simulink model "SG_GFOL_2020a"  (R2024a)
settings: Solver=ode1  StartTime=0.0  StopTime=Tsim  FixedStep=Ts  MaxStep=1e-4  RelTol=1e-4  EnableMultiTasking=on
values from neighbouring files (symbols this model uses):
  f1 = 50    [VSC_GF_SG_params.m]
  H = 5    [VSC_GF_SG_params.m]
  Inom_n2 = Sn_n2/Un_n2/sqrt(3)    [VSC_GF_SG_params.m]
  k_droop_f_n2 = 1/0.05    (= 20)    [VSC_GF_SG_params.m]
  ki_p_n2 = 1/tau_p    (= 5)    [VSC_GF_SG_params.m]
  ki_pll1 = kp_pll1/tau_pll_n1    [VSC_GF_SG_params.m]
  ki_pll_n2 = kp_pll_n2/tau_pll_n2    [VSC_GF_SG_params.m]
  ki_q_n2 = 1/tau_q    (= 5)    [VSC_GF_SG_params.m]
  ki_s_n2 = Rc_n2/taus_n2    (= 2048)    [VSC_GF_SG_params.m]
  kp_p_n2 = taus_n2/tau_p    (= 0.005)    [VSC_GF_SG_params.m]
  kp_pll1 = xi_pll_n1*2*omega_pll_n1/Vpeak    [VSC_GF_SG_params.m]
  kp_pll_n2 = xi_pll_n2*2*omega_pll_n2/Vpeak_n2    [VSC_GF_SG_params.m]
  kp_q_n2 = taus_n2/tau_q    (= 0.005)    [VSC_GF_SG_params.m]
  kp_s_n2 = Lc_n2/taus_n2    (= 130.379729381)    [VSC_GF_SG_params.m]
  Lac = Lpu*l*(Un1/Vl)^2    (= 0.105785123967)    [VSC_GF_SG_params.m]
  Lc_n2 = 0.2*Ln_n2    (= 0.130379729381)    [VSC_GF_SG_params.m]
  magnitud_delay = Ts    (= 5e-05)    [VSC_GF_SG_params.m]
  Pload_fnl = 400e6    (= 400000000)    [VSC_GF_SG_params.m]
  plots_step = Ts    (= 5e-05)    [VSC_GF_SG_params.m]
  Psg0_pu = Psg0/Pn    (= 0.4)    [VSC_GF_SG_params.m]
  Pvsc0 = Pload0 -Psg0    (= 200000000)    [VSC_GF_SG_params.m]
  Q_ref_n2 = 0e6    (= 0)    [VSC_GF_SG_params.m]
  Rac = Rpu*l*(Un1/Vl)^2    (= 3.17355371901)    [VSC_GF_SG_params.m]
  Rc_n2 = 0.01*Xn_n2    (= 2.048)    [VSC_GF_SG_params.m]
  Sn_n2 = Sn1    (= 500000000)    [VSC_GF_SG_params.m]
  Ssg = 500e6    (= 500000000)    [VSC_GF_SG_params.m]
  T_stp = 20    [VSC_GF_SG_params.m]
  tau_droop_fpll = 0.1    [VSC_GF_SG_params.m]
  tau_u = 40e-3    (= 0.04)    [VSC_GF_SG_params.m]
  Ts = 5e-5    (= 5e-05)    [VSC_GF_SG_params.m]
  Tsim = 40    [VSC_GF_SG_params.m]
  Un1 = 320e3    (= 320000)    [VSC_GF_SG_params.m]
  Vdcref_n1 = 640e3    (= 640000)    [VSC_GF_SG_params.m]
  Vpeak = Un1*sqrt(2/3)    [VSC_GF_SG_params.m]
  Vpeak_n1 = Un_n1/sqrt(3)*sqrt(2)    [VSC_GF_SG_params.m]
  Vpeak_n2 = Un_n2/sqrt(3)*sqrt(2)    [VSC_GF_SG_params.m]
  w_g1 = 2*pi*f1    (= 314.159265359)    [VSC_GF_SG_params.m]
  w_n2 = 2*pi*f_n2    (= 314.159265359)    [VSC_GF_SG_params.m]
undefined symbols (not defined in the file or in its folder): D11, Delta, k, magnitude, P_set, P_step, Pload_init, Q_set, Q_step, t_ramp, t_step_P, t_step_Q, tau_ramp, tau_wf
libraries: simulink x6, simulink_extras x6, spsSeriesRLCBranchLib x6, spsThreePhaseParallelRLCLoadLib x4, spsControlledVoltageSourceLib x4, spsCurrentMeasurementLib x4, spsControlledCurrentSourceLib x3, spsVoltageMeasurementLib x3, spsLoadFlowBusLib x2, slpidlib x2, spsGroundLib x2, spsSampleandHoldLib x1
(part 2 of 2)

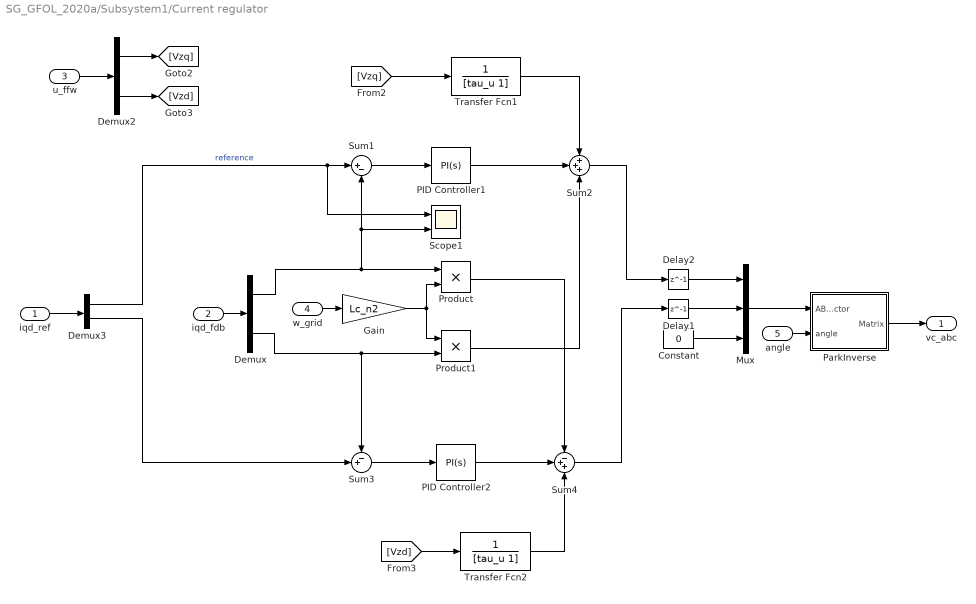
== system SG_GFOL_2020a/Subsystem1/Current regulator ==
  iqd_ref : Inport
  iqd_fdb : Inport  Port=2
  u_ffw : Inport  Port=3
  w_grid : Inport  Port=4
  angle : Inport  Port=5
  Constant : Constant  Value=0
  Delay1 : Delay  DelayLength=1  InitialCondition=0  SampleTime=magnitud_delay
  Delay2 : Delay  DelayLength=1  InitialCondition=Vpeak  SampleTime=magnitud_delay
  Demux : Demux  Outputs=2
  Demux2 : Demux  Outputs=2
  Demux3 : Demux  Outputs=2
  Gain : Gain  Gain=Lc_n2
  Mux : Mux  Inputs=3
  PID Controller1 : slpidlib/PID Controller  Controller=PI  Form=Parallel  TimeDomain=Continuous-time  UseExternalTs=off  SampleTime=-1  IntegratorMethod=Forward Euler  FilterMethod=Forward Euler  ControllerParametersSource=internal  P=kp_s_n2  I=ki_s_n2  UseKiTs=off  D=0  UseExternalDerivativeSource=off  N=100  UseFilter=on  TunerSelectOption=Transfer Function Based (PID Tuner App)  InitialConditionSource=internal  InitialConditionForIntegrator=0  InitialConditionForFilter=0  DifferentiatorICPrevScaledInput=0  ExternalReset=none  TrackingMode=off  Kt=1  LimitOutput=off  SatLimitsSource=internal  UpperSaturationLimit=inf  LowerSaturationLimit=-inf  LinearizeAsGain=on  AntiWindupMode=none  Kb=1  LimitIntegrator=off  UpperIntegratorSaturationLimit=inf  LowerIntegratorSaturationLimit=-inf  POutMin=[]  POutMax=[]  IOutMin=[]  IOutMax=[]  DOutMin=[]  DOutMax=[]  NOutMin=[]  NOutMax=[]  SumOutMin=[]  SumOutMax=[]  SaturationOutMin=[]  SaturationOutMax=[]  PParamMin=[]  PParamMax=[]  IParamMin=[]  IParamMax=[]  DParamMin=[]  DParamMax=[]  NParamMin=[]  NParamMax=[]  KbParamMin=[]  KbParamMax=[]  KtParamMin=[]  KtParamMax=[]  KbOutMin=[]  KbOutMax=[]  KtOutMin=[]  KtOutMax=[]  IntegratorOutMin=[]  IntegratorOutMax=[]  FilterOutMin=[]  FilterOutMax=[]  SumI1OutMin=[]  SumI1OutMax=[]  SumI2OutMin=[]  SumI2OutMax=[]  SumI3OutMin=[]  SumI3OutMax=[]  SumI4OutMin=[]  SumI4OutMax=[]  SumDOutMin=[]  SumDOutMax=[]  DifferentiatorOutMin=[]  DifferentiatorOutMax=[]  FilterDiffOutCoefMin=[]  FilterDiffOutCoefMax=[]  ReciprocalOutMin=[]  ReciprocalOutMax=[]  SumDenOutMin=[]  SumDenOutMax=[]  SumNumOutMin=[]  SumNumOutMax=[]  DivideOutMin=[]  DivideOutMax=[]  UdiffTsProdOutMin=[]  UdiffTsProdOutMax=[]  NTsProdOutMin=[]  NTsProdOutMax=[]  UintegralTsProdOutMin=[]  UintegralTsProdOutMax=[]  UngainTsProdOutMin=[]  UngainTsProdOutMax=[]  ClampingZeroOutDataTypeStr=Inherit: Inherit via back propagation  ClampingZeroOutMin=[]  ClampingZeroOutMax=[]  FilterDenConstantOutDataTypeStr=Inherit: Inherit via back propagation  FilterDenConstantOutMin=[]  FilterDenConstantOutMax=[]  PCopyOutDataTypeStr=Inherit: Inherit via back propagation  PCopyOutMin=[]  PCopyOutMax=[]  NCopyOutDataTypeStr=Inherit: Inherit via back propagation  NCopyOutMin=[]  NCopyOutMax=[]  IntegratorContinuousStateAttributes=''  IntegratorStateMustResolveToSignalObject=off  IntegratorRTWStateStorageClass=Auto  FilterContinuousStateAttributes=''  FilterStateMustResolveToSignalObject=off  FilterRTWStateStorageClass=Auto  ParallelPVariant=InternalParameters  IdealPVariant=Disabled  IVariant=InternalParameters  DVariant=Disabled  IntegratorVariant=Continuous  SatVariant=Disabled  AWVariant=Passthrough  PCopyVariant=Disabled  TRVariant=Disabled  FdbkBlocksVariant=Forward  IdealPFdbkVariant=Disabled  SatFdbkVariant=Disabled  DerivativeFilterVariant=Disabled  NVariant=Disabled  NCopyVariant=Disabled_SignalSpec  FilterICVariant=Disabled  IntegratorICVariant=InternalICs  ExternalResetVariant=Disabled  TRSumVariant=Passthrough  SumFdbkVariant=Disabled  SumVariant=Sum_PI  TsampFilterVariant=InternalTs  TsampNgainVariant=Passthrough  TsampIntegralVariant=Disabled_SignalSpec  ExternalSaturationOutDataTypeStr=Inherit: Same as second input  DerivativeSourceVariant=Disabled
  PID Controller2 : slpidlib/PID Controller  Controller=PI  Form=Parallel  TimeDomain=Continuous-time  UseExternalTs=off  SampleTime=-1  IntegratorMethod=Forward Euler  FilterMethod=Forward Euler  ControllerParametersSource=internal  P=kp_s_n2  I=ki_s_n2  UseKiTs=off  D=0  UseExternalDerivativeSource=off  N=100  UseFilter=on  TunerSelectOption=Transfer Function Based (PID Tuner App)  InitialConditionSource=internal  InitialConditionForIntegrator=0  InitialConditionForFilter=0  DifferentiatorICPrevScaledInput=0  ExternalReset=none  TrackingMode=off  Kt=1  LimitOutput=off  SatLimitsSource=internal  UpperSaturationLimit=inf  LowerSaturationLimit=-inf  LinearizeAsGain=on  AntiWindupMode=none  Kb=1  LimitIntegrator=off  UpperIntegratorSaturationLimit=inf  LowerIntegratorSaturationLimit=-inf  POutMin=[]  POutMax=[]  IOutMin=[]  IOutMax=[]  DOutMin=[]  DOutMax=[]  NOutMin=[]  NOutMax=[]  SumOutMin=[]  SumOutMax=[]  SaturationOutMin=[]  SaturationOutMax=[]  PParamMin=[]  PParamMax=[]  IParamMin=[]  IParamMax=[]  DParamMin=[]  DParamMax=[]  NParamMin=[]  NParamMax=[]  KbParamMin=[]  KbParamMax=[]  KtParamMin=[]  KtParamMax=[]  KbOutMin=[]  KbOutMax=[]  KtOutMin=[]  KtOutMax=[]  IntegratorOutMin=[]  IntegratorOutMax=[]  FilterOutMin=[]  FilterOutMax=[]  SumI1OutMin=[]  SumI1OutMax=[]  SumI2OutMin=[]  SumI2OutMax=[]  SumI3OutMin=[]  SumI3OutMax=[]  SumI4OutMin=[]  SumI4OutMax=[]  SumDOutMin=[]  SumDOutMax=[]  DifferentiatorOutMin=[]  DifferentiatorOutMax=[]  FilterDiffOutCoefMin=[]  FilterDiffOutCoefMax=[]  ReciprocalOutMin=[]  ReciprocalOutMax=[]  SumDenOutMin=[]  SumDenOutMax=[]  SumNumOutMin=[]  SumNumOutMax=[]  DivideOutMin=[]  DivideOutMax=[]  UdiffTsProdOutMin=[]  UdiffTsProdOutMax=[]  NTsProdOutMin=[]  NTsProdOutMax=[]  UintegralTsProdOutMin=[]  UintegralTsProdOutMax=[]  UngainTsProdOutMin=[]  UngainTsProdOutMax=[]  ClampingZeroOutDataTypeStr=Inherit: Inherit via back propagation  ClampingZeroOutMin=[]  ClampingZeroOutMax=[]  FilterDenConstantOutDataTypeStr=Inherit: Inherit via back propagation  FilterDenConstantOutMin=[]  FilterDenConstantOutMax=[]  PCopyOutDataTypeStr=Inherit: Inherit via back propagation  PCopyOutMin=[]  PCopyOutMax=[]  NCopyOutDataTypeStr=Inherit: Inherit via back propagation  NCopyOutMin=[]  NCopyOutMax=[]  IntegratorContinuousStateAttributes=''  IntegratorStateMustResolveToSignalObject=off  IntegratorRTWStateStorageClass=Auto  FilterContinuousStateAttributes=''  FilterStateMustResolveToSignalObject=off  FilterRTWStateStorageClass=Auto  ParallelPVariant=InternalParameters  IdealPVariant=Disabled  IVariant=InternalParameters  DVariant=Disabled  IntegratorVariant=Continuous  SatVariant=Disabled  AWVariant=Passthrough  PCopyVariant=Disabled  TRVariant=Disabled  FdbkBlocksVariant=Forward  IdealPFdbkVariant=Disabled  SatFdbkVariant=Disabled  DerivativeFilterVariant=Disabled  NVariant=Disabled  NCopyVariant=Disabled_SignalSpec  FilterICVariant=Disabled  IntegratorICVariant=InternalICs  ExternalResetVariant=Disabled  TRSumVariant=Passthrough  SumFdbkVariant=Disabled  SumVariant=Sum_PI  TsampFilterVariant=InternalTs  TsampNgainVariant=Passthrough  TsampIntegralVariant=Disabled_SignalSpec  ExternalSaturationOutDataTypeStr=Inherit: Same as second input  DerivativeSourceVariant=Disabled
  ParkInverse : Subsystem  mask(Gerard){}
      mask help:
      | This block applies the park inverse transfomation from a desired vector.
      | The input Xqd0 refers to the vector in the qd0 frame, and the second input is the angle used in the inverse transformation.
      | The output is the vector in the ABC frame.
      mask Display:
      | port_label('output',1,'Xabc')
      | port_label('input',1,'Xqd0')
      | port_label('input',2,'angle')
  Product : Product  RndMeth=Zero
  Product1 : Product  RndMeth=Zero
  Scope1 : Scope  NumInputPorts=2
  Sum1 : Sum  Inputs=|+-
  Sum2 : Sum  Inputs=+++
  Sum3 : Sum  Inputs=-+|
  Sum4 : Sum  Inputs=-++
  Transfer Fcn1 : TransferFcn  Denominator=[tau_u 1]
  Transfer Fcn2 : TransferFcn  Denominator=[tau_u 1]
  vc_abc : Outport
  wires:
  Transfer Fcn2/1 -> Sum4/3
  [Vzq] -> Transfer Fcn1/1
  Demux3/2 -> Sum3/2
  iqd_ref/1 -> Demux3/1
  Demux3/1 -> Scope1/1, Sum1/1  "reference"
  PID Controller2/1 -> Sum4/2
  Sum3/1 -> PID Controller2/1
  Sum1/1 -> PID Controller1/1
  angle/1 -> ParkInverse/2(angle)
  [Vzd] -> Transfer Fcn2/1
  u_ffw/1 -> Demux2/1
  Demux2/2 -> [Vzd]
  Demux2/1 -> [Vzq]
  Mux/1 -> ParkInverse/1(ABC vector)
  Transfer Fcn1/1 -> Sum2/1
  ParkInverse/1(Matrix) -> vc_abc/1
  Constant/1 -> Mux/3
  Product/1 -> Sum4/1
  Product1/1 -> Sum2/3
  Demux/2 -> Sum3/1, Product1/2
  Gain/1 -> Product/2, Product1/1
  Demux/1 -> Product/1, Scope1/2, Sum1/2
  PID Controller1/1 -> Sum2/2
  w_grid/1 -> Gain/1
  iqd_fdb/1 -> Demux/1
  Sum4/1 -> Delay1/1
  Sum2/1 -> Delay2/1
  Delay1/1 -> Mux/2
  Delay2/1 -> Mux/1

== system SG_GFOL_2020a/Subsystem1/Frequency support ==
  wref : Inport
  wpll : Inport  Port=2
  Pref0 : Inport  Port=3
  Gain1 : Gain  Gain=Sn_n2
  Gain10 : Gain  Gain=1/w_n2
  Product : Product
  Sum2 : Sum  Inputs=|+-
  Sum3 : Sum  Inputs=|++
  Transfer Fcn2 : TransferFcn  Denominator=[tau_droop_fpll 1]
  kdroop : Step  After=k_droop_f_n2  SampleTime=0
  Pref : Outport
  wires:
  Gain1/1 -> Sum3/1
  Gain10/1 -> Product/1
  Transfer Fcn2/1 -> Sum2/2
  kdroop/1 -> Product/2
  Product/1 -> Gain1/1
  wpll/1 -> Transfer Fcn2/1
  Sum3/1 -> Pref/1
  Pref0/1 -> Sum3/2
  Sum2/1 -> Gain10/1
  wref/1 -> Sum2/1

== system SG_GFOL_2020a/Subsystem1/PLL ==
  Vabc : Inport
  Constant1 : Constant  Value=w_n2
  Demux3 : Demux  Outputs=3
  Integrator2 : Integrator
  Integrator3 : Integrator
  Mux : Mux  Inputs=2
  ParkTransform4 : Subsystem  mask(Gerard){}
      mask help:
      | This block applies the park transfomation from a desired vector.
      | The input Xabc refers to the vector in the ABC frame, and the second input is the angle used in the transformation.
      | The output is the vector in the qd0 frame.
      mask Display:
      | port_label('output',1,'Xqd0')
      | port_label('input',1,'Xabc')
      | port_label('input',2,'angle')
  Sum1 : Sum  Inputs=+++
  Terminator : Terminator
  ki1 : Gain  Gain=ki_pll_n2
  kp1 : Gain  Gain=-1
  kp2 : Gain  Gain=kp_pll_n2
  omega : Outport  VectorParamsAs1DForOutWhenUnconnected=off
  angle : Outport  Port=2  VectorParamsAs1DForOutWhenUnconnected=off
  vqd : Outport  Port=3  VectorParamsAs1DForOutWhenUnconnected=off
  wires:
  Sum1/1 -> omega/1, Integrator3/1
  Demux3/1 -> Mux/1
  Constant1/1 -> Sum1/1
  ki1/1 -> Integrator2/1
  kp1/1 -> kp2/1, ki1/1
  Integrator2/1 -> Sum1/3
  kp2/1 -> Sum1/2
  Integrator3/1 -> ParkTransform4/2(angle), angle/1
  Demux3/2 -> Mux/2, kp1/1  "Vd"
  Vabc/1 -> ParkTransform4/1(ABC vector)
  ParkTransform4/1(Matrix) -> Demux3/1
  Demux3/3 -> Terminator/1
  Mux/1 -> vqd/1

== system SG_GFOL_2020a/Subsystem1/PQ Calculation1 ==
  u_qd : Inport
  ig_qd : Inport  Port=2
  Add1 : Sum  Inputs=-+
  Add2 : Sum
  Demux4 : Demux  Outputs=2
  Demux7 : Demux  Outputs=2
  Gain1 : Gain  Gain=3/2
  Gain12 : Gain  Gain=3/2
  Product{,1..3} (4 alike) : Product
  P : Outport
  Q : Outport  Port=2
  wires:
  Gain12/1 -> P/1
  Gain1/1 -> Q/1
  u_qd/1 -> Demux7/1
  ig_qd/1 -> Demux4/1
  Product3/1 -> Add1/2
  Add1/1 -> Gain1/1
  Demux4/1 -> Product/2, Product2/2
  Product2/1 -> Add1/1
  Demux7/1 -> Product/1, Product3/1
  Add2/1 -> Gain12/1
  Product1/1 -> Add2/2
  Product/1 -> Add2/1
  Demux7/2 -> Product1/1, Product2/1
  Demux4/2 -> Product3/2, Product1/2

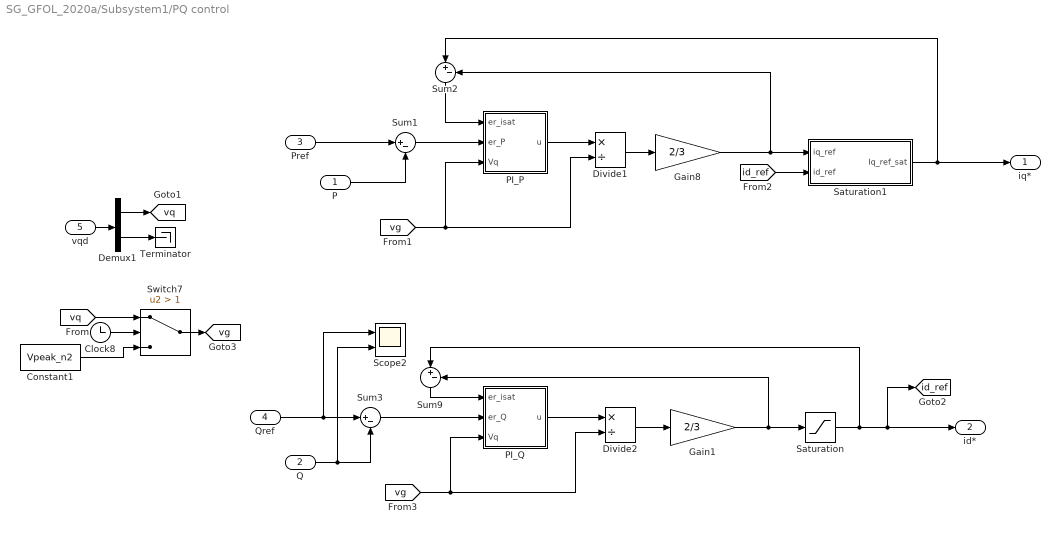
== system SG_GFOL_2020a/Subsystem1/PQ control ==
  P : Inport
  Q : Inport  Port=2
  Pref : Inport  Port=3
  Qref : Inport  Port=4
  vqd : Inport  Port=5
  Clock8 : Clock
  Constant1 : Constant  Value=Vpeak_n2
  Demux1 : Demux  Outputs=2
  Divide1 : Product  Inputs=*/
  Divide2 : Product  Inputs=*/
  Gain1 : Gain  Gain=2/3
  Gain8 : Gain  Gain=2/3
  PI_P : Subsystem
  PI_Q : Subsystem
  Saturation : Saturate  UpperLimit=Inom_n2  LowerLimit=-Inom_n2
  Saturation1 : Subsystem
  Scope2 : Scope  NumInputPorts=2
  Sum{1..3,9} (4 alike) : Sum  Inputs=|+-
  Switch7 : Switch  Criteria=u2 > Threshold  Threshold=1  SaturateOnIntegerOverflow=off  InputSameDT=off
  Terminator : Terminator
  iq* : Outport
  id* : Outport  Port=2
  tag scope: id_ref=global, vg=global, vq=global
  wires:
  Gain1/1 -> Sum9/2, Saturation/1
  Pref/1 -> Sum1/1
  Sum3/1 -> PI_Q/2(er_Q)
  Qref/1 -> Scope2/1, Sum3/1
  P/1 -> Sum1/2
  Q/1 -> Scope2/2, Sum3/2
  [vg] -> Divide1/2, PI_P/3(Vq)
  PI_P/1(u) -> Divide1/1
  Gain8/1 -> Sum2/2, Saturation1/1(iq_ref)
  Saturation1/1(Iq_ref_sat) -> Sum2/1, iq*/1
  Divide1/1 -> Gain8/1
  Sum1/1 -> PI_P/2(er_P)
  vqd/1 -> Demux1/1
  Demux1/2 -> Terminator/1
  PI_Q/1(u) -> Divide2/1
  Divide2/1 -> Gain1/1
  Demux1/1 -> [vq]
  [vg] -> PI_Q/3(Vq), Divide2/2
  Saturation/1 -> [id_ref], id*/1, Sum9/1
  Sum9/1 -> PI_Q/1(er_isat)
  Sum2/1 -> PI_P/1(er_isat)
  [id_ref] -> Saturation1/2(id_ref)
  [vq] -> Switch7/1
  Constant1/1 -> Switch7/3
  Clock8/1 -> Switch7/2
  Switch7/1 -> [vg]

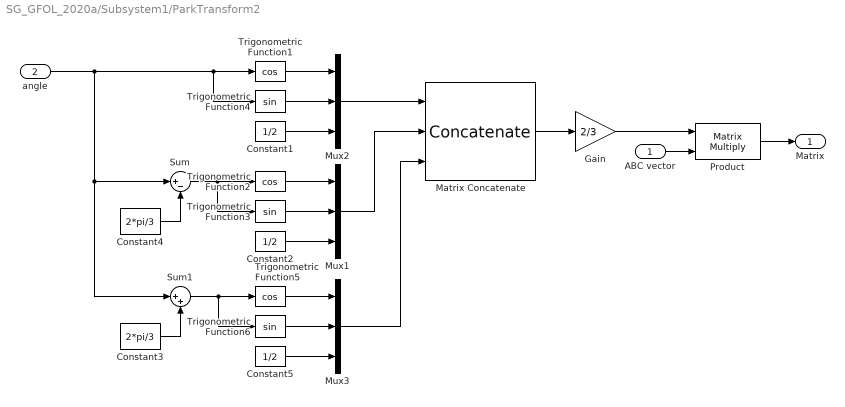
== system SG_GFOL_2020a/Subsystem1/ParkTransform2 ==
  ABC vector : Inport
  angle : Inport  Port=2
  Constant1 : Constant  Value=1/2
  Constant2 : Constant  Value=1/2
  Constant3 : Constant  Value=2*pi/3
  Constant4 : Constant  Value=2*pi/3
  Constant5 : Constant  Value=1/2
  Gain : Gain  Gain=2/3
  Matrix Concatenate : Concatenate  NumInputs=3  Mode=Multidimensional array  ConcatenateDimension=2
  Mux1 : Mux  Inputs=3
  Mux2 : Mux  Inputs=3
  Mux3 : Mux  Inputs=3
  Product : Product  Multiplication=Matrix(*)  RndMeth=Zero
  Sum : Sum  Inputs=|+-
  Sum1 : Sum  Inputs=|++
  Trigonometric Function1 : Trigonometry  Operator=cos
  Trigonometric Function2 : Trigonometry  Operator=cos
  Trigonometric Function3 : Trigonometry
  Trigonometric Function4 : Trigonometry
  Trigonometric Function5 : Trigonometry  Operator=cos
  Trigonometric Function6 : Trigonometry
  Matrix : Outport
  wires:
  Mux3/1 -> Matrix Concatenate/3
  Mux2/1 -> Matrix Concatenate/1
  Mux1/1 -> Matrix Concatenate/2
  Sum1/1 -> Trigonometric Function5/1, Trigonometric Function6/1
  Constant5/1 -> Mux3/3
  Trigonometric Function5/1 -> Mux3/1
  Trigonometric Function6/1 -> Mux3/2
  Constant1/1 -> Mux2/3
  Trigonometric Function1/1 -> Mux2/1
  Trigonometric Function4/1 -> Mux2/2
  Sum/1 -> Trigonometric Function2/1, Trigonometric Function3/1
  Constant2/1 -> Mux1/3
  Trigonometric Function2/1 -> Mux1/1
  Trigonometric Function3/1 -> Mux1/2
  angle/1 -> Sum/1, Sum1/1, Trigonometric Function1/1, Trigonometric Function4/1
  Constant3/1 -> Sum1/2
  Constant4/1 -> Sum/2
  Gain/1 -> Product/1
  Product/1 -> Matrix/1
  ABC vector/1 -> Product/2
  Matrix Concatenate/1 -> Gain/1

== system SG_GFOL_2020a/Subsystem1/VSC n1 ==
  vc_abc : Inport
  i_abc : Inport  Port=2
  Vbus : Inport  Port=3
  Controlled Current Source5 : spsControlledCurrentSourceLib/Controlled Current Source  Initialize=on  Source_Type=DC  Amplitude=0  Phase=0  Frequency=0  Measurements=None
  Controlled Voltage Source1 : spsControlledVoltageSourceLib/Controlled Voltage Source  Initialize=off  Source_Type=AC  Amplitude=0  Phase=0  Frequency=0  Measurements=None
  Controlled Voltage Source2 : spsControlledVoltageSourceLib/Controlled Voltage Source  Initialize=off  Source_Type=AC  Amplitude=0  Phase=0  Frequency=0  Measurements=None
  Controlled Voltage Source3 : spsControlledVoltageSourceLib/Controlled Voltage Source  Initialize=off  Source_Type=AC  Amplitude=0  Phase=0  Frequency=0  Measurements=None
  Current Measurement9 : spsCurrentMeasurementLib/Current Measurement  PhasorSimulation=off  OutputType=Complex  PSBequivalent=0
  Demux : Demux  Outputs=3
  Divide : Product  Inputs=*/
  Ground : spsGroundLib/Ground  LConnTagsString=a
  Product1 : Product  InputSameDT=on  SaturateOnIntegerOverflow=on  OutDataTypeStr=Inherit: Same as first input
  Sum4 : Sum  Inputs=1  InputSameDT=on  SaturateOnIntegerOverflow=on  OutDataTypeStr=Inherit: Same as first input
  vc_abc1 : InportShadow
  a : PMIOPort  Side=Left
  b : PMIOPort  Port=2  Side=Left
  c : PMIOPort  Port=3  Side=Left
  DC+ : PMIOPort  Port=4  Side=Right
  DC- : PMIOPort  Port=5  Side=Right
  idc : Outport
  wires:
  Vbus/1 -> Divide/2
  vc_abc/1 -> Demux/1
  Demux/3 -> Controlled Voltage Source3/1
  Demux/1 -> Controlled Voltage Source1/1
  Demux/2 -> Controlled Voltage Source2/1
  i_abc/1 -> Product1/2
  vc_abc1/1 -> Product1/1
  Divide/1 -> Controlled Current Source5/1
  Sum4/1 -> Divide/1
  Product1/1 -> Sum4/1
  Current Measurement9/1 -> idc/1
  connections:
  c/RConn1 -- Controlled Voltage Source3/RConn1
  b/RConn1 -- Controlled Voltage Source2/RConn1
  a/RConn1 -- Controlled Voltage Source1/RConn1
  Controlled Voltage Source3/LConn1 -- Ground/LConn1 -- Controlled Voltage Source2/LConn1 -- Controlled Voltage Source1/LConn1
  Current Measurement9/LConn1 -- DC+/RConn1
  Controlled Current Source5/LConn1 -- Current Measurement9/RConn1
  Controlled Current Source5/RConn1 -- DC-/RConn1

== system SG_GFOL_2020a/Subsystem1/Virtual inertia ==
  wpll : Inport
  Pref0 : Inport  Port=2
  Gain1 : Gain  Gain=k
  Integrator : Integrator
  Sum2 : Sum  Inputs=|+-
  Sum3 : Sum  Inputs=|++
  Transfer Fcn2 : TransferFcn  Denominator=[tau_droop_fpll 1]
  Pref : Outport
  wires:
  Transfer Fcn2/1 -> Integrator/1, Sum2/1
  wpll/1 -> Transfer Fcn2/1
  Pref0/1 -> Sum3/2
  Sum2/1 -> Gain1/1
  Sum3/1 -> Pref/1
  Integrator/1 -> Sum2/2
  Gain1/1 -> Sum3/1

== system SG_GFOL_2020a/G1/Exciter System/PSS1 ==
  note: Power System Stabilizer (PSS2A)
  dw : Inport
  Pgen : Inport  Port=2
  Gain : Gain  Gain=Ks1
  Gain1 : Gain  Gain=Ks3
  Saturation : Saturate  UpperLimit=Vstmax  LowerLimit=Vstmin
  Sum1 : Sum  Inputs=|++
  Sum2 : Sum  Inputs=|+-
  Transfer Fcn1 : TransferFcn  Numerator=[Tw1 0]  Denominator=[Tw1 1]
  Transfer Fcn2 : TransferFcn  Numerator=[Tw3 0]  Denominator=[Tw3 1]
  Transfer Fcn3 : TransferFcn  Numerator=[Tw2 0]  Denominator=[Tw2 1]
  Transfer Fcn4 : TransferFcn  Denominator=[T6 1]
  Transfer Fcn5 : TransferFcn  Numerator=[T8 1].^N  Denominator=[T9 1].^(M*N)
  Transfer Fcn6 : TransferFcn  Numerator=[T1 1]  Denominator=[T2 1]
  Transfer Fcn7 : TransferFcn  Numerator=[T3 1]  Denominator=[T4 1]
  Transfer Fcn8 : TransferFcn  Numerator=[Tw4 0]  Denominator=[Tw4 1]
  Transfer Fcn9 : TransferFcn  Numerator=[Ks2]  Denominator=[T7 1]
  Vothsg : Outport
  wires:
  dw/1 -> Transfer Fcn1/1
  Transfer Fcn1/1 -> Transfer Fcn3/1
  Transfer Fcn3/1 -> Transfer Fcn4/1
  Transfer Fcn4/1 -> Sum1/1
  Sum1/1 -> Transfer Fcn5/1
  Transfer Fcn5/1 -> Sum2/1
  Sum2/1 -> Gain/1
  Gain/1 -> Transfer Fcn6/1
  Transfer Fcn6/1 -> Transfer Fcn7/1
  Transfer Fcn7/1 -> Saturation/1
  Saturation/1 -> Vothsg/1
  Pgen/1 -> Transfer Fcn2/1
  Transfer Fcn2/1 -> Transfer Fcn8/1
  Transfer Fcn8/1 -> Transfer Fcn9/1
  Gain1/1 -> Sum1/2
  Transfer Fcn9/1 -> Gain1/1, Sum2/2

== system SG_GFOL_2020a/G1/Exciter System/PSS1 backup ==
  note: Power System Stabilizer (PSS2A)
  dw : Inport
  Pgen : Inport  Port=2
  Gain : Gain  Gain=Ks1
  Gain1 : Gain  Gain=Ks3
  Saturation : Saturate  UpperLimit=Vstmax  LowerLimit=Vstmin
  Sum1 : Sum  Inputs=|++
  Sum2 : Sum  Inputs=|+-
  Transfer Fcn1 : TransferFcn  Numerator=[Tw1 0]  Denominator=[Tw1 1]
  Transfer Fcn2 : TransferFcn  Numerator=[Tw3 0]  Denominator=[Tw3 1]
  Transfer Fcn3 : TransferFcn  Numerator=[Tw2 0]  Denominator=[Tw2 1]
  Transfer Fcn4 : TransferFcn  Denominator=[T6 1]
  Transfer Fcn5 : TransferFcn  Numerator=[T8 1].^N  Denominator=[T9 1].^(M*N)
  Transfer Fcn6 : TransferFcn  Numerator=[T1 1]  Denominator=[T2 1]
  Transfer Fcn7 : TransferFcn  Numerator=[T3 1]  Denominator=[T4 1]
  Transfer Fcn8 : TransferFcn  Numerator=[Tw4 0]  Denominator=[Tw4 1]
  Transfer Fcn9 : TransferFcn  Numerator=[Ks2]  Denominator=[T7 1]
  Vothsg : Outport
  wires:
  Transfer Fcn9/1 -> Sum2/2, Gain1/1
  Gain1/1 -> Sum1/2
  Transfer Fcn8/1 -> Transfer Fcn9/1
  Transfer Fcn2/1 -> Transfer Fcn8/1
  Pgen/1 -> Transfer Fcn2/1
  Saturation/1 -> Vothsg/1
  Transfer Fcn7/1 -> Saturation/1
  Transfer Fcn6/1 -> Transfer Fcn7/1
  Gain/1 -> Transfer Fcn6/1
  Sum2/1 -> Gain/1
  Transfer Fcn5/1 -> Sum2/1
  Sum1/1 -> Transfer Fcn5/1
  Transfer Fcn4/1 -> Sum1/1
  Transfer Fcn3/1 -> Transfer Fcn4/1
  Transfer Fcn1/1 -> Transfer Fcn3/1
  dw/1 -> Transfer Fcn1/1

== system SG_GFOL_2020a/G1/Exciter System/SEXS ==
  note: The controller parameters provided by ENTSO-E
      | define different names for the parameters:
      |
      | ENTSO-E = IEEE Std 421.5-2005
      | Ta = Tc
      | Tb = Tb
      | K = Ka
      | Te = Ta
      | Emax = Vrmax
      | Emin = Vrmin
  note: The exciter model provided by ENTSO-E most similar to the IEEE is the Type AC4A excitation system model
  Vref : Inport
  Vc : Inport  Port=2
  Vs : Inport  Port=3
  1st ord transfer fcn windup limiter : Subsystem  mask{Gain=K, tau=Te, Vmax=Emax, Vmin=Emin, y0=Vf0}
      mask prompts: tau "Time constant"; y0 "Initial output"
  Constant : Constant  Value=Vf0/K
  Saturation : Saturate  Commented=through  UpperLimit=0.1  LowerLimit=-0.1
  Sum : Sum  Inputs=+-+
  Sum1 : Sum  Inputs=|++
  Transfer Fcn (with initial outputs)1 : simulink_extras/Additional Linear/Transfer Fcn (with initial outputs)  N=[Ta 1]  D=[Tb 1]  Y0=Vf0/K  U0=Vf0/K
  Efd : Outport
  wires:
  1st ord transfer fcn windup limiter/1(Out1) -> Efd/1
  Vs/1 -> Sum/3
  Vref/1 -> Sum/1
  Vc/1 -> Sum/2
  Transfer Fcn (with initial outputs)1/1 -> 1st ord transfer fcn windup limiter/1(In1)
  Saturation/1 -> Transfer Fcn (with initial outputs)1/1
  Sum/1 -> Sum1/1
  Sum1/1 -> Saturation/1
  Constant/1 -> Sum1/2

== system SG_GFOL_2020a/G1/Exciter System/TR and LC_test ==
  note: Terminal voltage transducer and optional load compensation
  note: compensated
      | impedance
  note: Vt and It should be phasors (complex quantities)
  note: Fig 4.1 of IEEE Std 421.5-2005
  note: Rc and Xc should be negative values in case of voltage regulated after an impedance
  Vt : Inport
  It : Inport  Port=2
  Abs : Abs  SaturateOnIntegerOverflow=off
  Abs1 : Abs  SaturateOnIntegerOverflow=off
  Rc+jXc : Gain  Gain=abs(Rc+1i*Xc)
  Saturation : Saturate  UpperLimit=1.2  LowerLimit=0.8
  Sum : Sum  Inputs=|+-
  Transfer Fcn (with initial outputs) : simulink_extras/Additional Linear/Transfer Fcn (with initial outputs)  Commented=through  N=[1]  D=[Tr 1]  Y0=1  U0=1
  Vc : Outport
  wires:
  Saturation/1 -> Vc/1
  Vt/1 -> Abs/1
  Transfer Fcn (with initial outputs)/1 -> Saturation/1
  Rc+jXc/1 -> Sum/2
  Sum/1 -> Transfer Fcn (with initial outputs)/1
  It/1 -> Abs1/1
  Abs/1 -> Sum/1
  Abs1/1 -> Rc+jXc/1

== system SG_GFOL_2020a/Other blocks (do not use)/PQ/PLL ==
  u_abc : Inport
  Constant : Constant  Value=0
  Constant3 : Constant  Value=2*pi*f1
  Constant4 : Constant  Value=2*pi
  Demux : Demux  Outputs=3
  Integrator : Integrator
  Math Function : Math  Operator=mod  SignedPower=on
  PID Controller : simulink/Continuous/PID Controller  Controller=PI  Form=Parallel  TimeDomain=Continuous-time  UseExternalTs=off  SampleTime=-1  IntegratorMethod=Forward Euler  FilterMethod=Forward Euler  ControllerParametersSource=internal  P=kp_pll1  I=ki_pll1  D=0  UseFilter=on  N=100  TunerSelectOption=Transfer Function Based (PID Tuner App)  InitialConditionSource=internal  InitialConditionForIntegrator=0  InitialConditionForFilter=0  DifferentiatorICPrevScaledInput=0  ExternalReset=none  TrackingMode=off  Kt=1  LimitOutput=off  UpperSaturationLimit=inf  LowerSaturationLimit=-inf  LinearizeAsGain=on  AntiWindupMode=none  Kb=1  POutMin=[]  POutMax=[]  IOutMin=[]  IOutMax=[]  DOutMin=[]  DOutMax=[]  NOutMin=[]  NOutMax=[]  SumOutMin=[]  SumOutMax=[]  SaturationOutMin=[]  SaturationOutMax=[]  PParamMin=[]  PParamMax=[]  IParamMin=[]  IParamMax=[]  DParamMin=[]  DParamMax=[]  NParamMin=[]  NParamMax=[]  KbParamMin=[]  KbParamMax=[]  KtParamMin=[]  KtParamMax=[]  KbOutMin=[]  KbOutMax=[]  KtOutMin=[]  KtOutMax=[]  IntegratorOutMin=[]  IntegratorOutMax=[]  FilterOutMin=[]  FilterOutMax=[]  SumI1OutMin=[]  SumI1OutMax=[]  SumI2OutMin=[]  SumI2OutMax=[]  SumI3OutMin=[]  SumI3OutMax=[]  SumI4OutMin=[]  SumI4OutMax=[]  SumDOutMin=[]  SumDOutMax=[]  DifferentiatorOutMin=[]  DifferentiatorOutMax=[]  FilterDiffOutCoefMin=[]  FilterDiffOutCoefMax=[]  ReciprocalOutMin=[]  ReciprocalOutMax=[]  SumDenOutMin=[]  SumDenOutMax=[]  SumNumOutMin=[]  SumNumOutMax=[]  DivideOutMin=[]  DivideOutMax=[]  UdiffTsProdOutMin=[]  UdiffTsProdOutMax=[]  NTsProdOutMin=[]  NTsProdOutMax=[]  UintegralTsProdOutMin=[]  UintegralTsProdOutMax=[]  UngainTsProdOutMin=[]  UngainTsProdOutMax=[]  IntegratorContinuousStateAttributes=''  IntegratorStateMustResolveToSignalObject=off  IntegratorRTWStateStorageClass=Auto  FilterContinuousStateAttributes=''  FilterStateMustResolveToSignalObject=off  FilterRTWStateStorageClass=Auto  ParallelPVariant=InternalParameters  IdealPVariant=Disabled  IVariant=InternalParameters  DVariant=Disabled  IntegratorVariant=Continuous  SatVariant=Disabled  AWVariant=Passthrough  PCopyVariant=Disabled  TRVariant=Disabled  FdbkBlocksVariant=Forward  IdealPFdbkVariant=Disabled  SatFdbkVariant=Disabled  DerivativeFilterVariant=Disabled  NVariant=Disabled  NCopyVariant=Disabled_SignalSpec  FilterICVariant=Disabled  IntegratorICVariant=InternalICs  ExternalResetVariant=Disabled  TRSumVariant=Passthrough  SumFdbkVariant=Disabled  SumVariant=Sum_PI  TsampFilterVariant=InternalTs  TsampNgainVariant=Passthrough  TsampIntegralVariant=Passthrough
  ParkTransform7 : Subsystem  mask(Gerard){}
      mask help:
      | This block applies the park transfomation from a desired vector.
      | The input Xabc refers to the vector in the ABC frame, and the second input is the angle used in the transformation.
      | The output is the vector in the qd0 frame.
      mask Display:
      | port_label('output',1,'Xqd0')
      | port_label('input',1,'Xabc')
      | port_label('input',2,'angle')
  Scope1 : Scope
  Scope20 : Scope
  Sum : Sum  Inputs=|+-
  Sum1 : Sum  Inputs=|++
  Terminator8 : Terminator
  Vzq : Outport
  Vzd : Outport  Port=2
  angle : Outport  Port=3
  w_grid : Outport  Port=4
  wires:
  Math Function/1 -> Scope1/1
  Demux/1 -> Vzq/1
  Sum/1 -> PID Controller/1, Scope20/1
  ParkTransform7/1(Matrix) -> Demux/1
  u_abc/1 -> ParkTransform7/1(ABC vector)
  PID Controller/1 -> Sum1/1
  Demux/3 -> Terminator8/1
  Integrator/1 -> angle/1, Math Function/1, ParkTransform7/2(angle)
  Constant4/1 -> Math Function/2
  Constant/1 -> Sum/1
  Sum1/1 -> Integrator/1, w_grid/1
  Demux/2 -> Sum/2, Vzd/1
  Constant3/1 -> Sum1/2

== system SG_GFOL_2020a/Other blocks (do not use)/PQ/ParkInverse1 ==
  ABC vector : Inport
  angle : Inport  Port=2
  Constant4 : Constant  Value=2*pi/3
  Constant5 : Constant  Value=2*pi/3
  Constant9 : Constant
  Matrix Concatenate2 : Concatenate  NumInputs=3  Mode=Multidimensional array  ConcatenateDimension=2
  Mux6 : Mux  Inputs=3
  Mux7 : Mux  Inputs=3
  Product : Product  Multiplication=Matrix(*)  RndMeth=Zero
  Signal Specification1 : SignalSpecification  Dimensions=3
  Signal Specification4 : SignalSpecification  Dimensions=3
  Sum : Sum  Inputs=|+-
  Sum1 : Sum  Inputs=|++
  Trigonometric Function8 : Trigonometry  Operator=cos
  Trigonometric Function9 : Trigonometry
  Matrix : Outport
  wires:
  Signal Specification1/1 -> Matrix Concatenate2/2
  Signal Specification4/1 -> Matrix Concatenate2/1
  angle/1 -> Sum1/1, Sum/1, Mux6/1
  Constant5/1 -> Sum1/2
  Constant4/1 -> Sum/2
  Product/1 -> Matrix/1
  ABC vector/1 -> Product/2
  Sum/1 -> Mux6/2
  Sum1/1 -> Mux6/3
  Constant9/1 -> Mux7/3, Mux7/1, Mux7/2
  Trigonometric Function8/1 -> Signal Specification4/1
  Trigonometric Function9/1 -> Signal Specification1/1
  Mux6/1 -> Trigonometric Function9/1, Trigonometric Function8/1
  Mux7/1 -> Matrix Concatenate2/3
  Matrix Concatenate2/1 -> Product/1

== system SG_GFOL_2020a/Subsystem1/Current regulator/ParkInverse ==
  ABC vector : Inport
  angle : Inport  Port=2
  Constant4 : Constant  Value=2*pi/3
  Constant5 : Constant  Value=2*pi/3
  Constant9 : Constant
  Matrix Concatenate2 : Concatenate  NumInputs=3  Mode=Multidimensional array  ConcatenateDimension=2
  Mux6 : Mux  Inputs=3
  Mux7 : Mux  Inputs=3
  Product : Product  Multiplication=Matrix(*)  RndMeth=Zero
  Sum : Sum  Inputs=|+-
  Sum1 : Sum  Inputs=|++
  Trigonometric Function8 : Trigonometry  Operator=cos
  Trigonometric Function9 : Trigonometry
  Matrix : Outport
  wires:
  Matrix Concatenate2/1 -> Product/1
  Mux7/1 -> Matrix Concatenate2/3
  Mux6/1 -> Trigonometric Function8/1, Trigonometric Function9/1
  Trigonometric Function9/1 -> Matrix Concatenate2/2
  Trigonometric Function8/1 -> Matrix Concatenate2/1
  Constant9/1 -> Mux7/2, Mux7/1, Mux7/3
  Sum1/1 -> Mux6/3
  Sum/1 -> Mux6/2
  ABC vector/1 -> Product/2
  Product/1 -> Matrix/1
  Constant4/1 -> Sum/2
  Constant5/1 -> Sum1/2
  angle/1 -> Mux6/1, Sum/1, Sum1/1

== system SG_GFOL_2020a/Subsystem1/PLL/ParkTransform4 ==
  ABC vector : Inport
  angle : Inport  Port=2
  Constant1 : Constant  Value=1/2
  Constant2 : Constant  Value=1/2
  Constant3 : Constant  Value=2*pi/3
  Constant4 : Constant  Value=2*pi/3
  Constant5 : Constant  Value=1/2
  Gain : Gain  Gain=2/3
  Matrix Concatenate : Concatenate  NumInputs=3  Mode=Multidimensional array  ConcatenateDimension=2
  Mux1 : Mux  Inputs=3
  Mux2 : Mux  Inputs=3
  Mux3 : Mux  Inputs=3
  Product : Product  Multiplication=Matrix(*)  RndMeth=Zero
  Sum : Sum  Inputs=|+-
  Sum1 : Sum  Inputs=|++
  Trigonometric Function1 : Trigonometry  Operator=cos
  Trigonometric Function2 : Trigonometry  Operator=cos
  Trigonometric Function3 : Trigonometry
  Trigonometric Function4 : Trigonometry
  Trigonometric Function5 : Trigonometry  Operator=cos
  Trigonometric Function6 : Trigonometry
  Matrix : Outport
  wires:
  Matrix Concatenate/1 -> Gain/1
  ABC vector/1 -> Product/2
  Product/1 -> Matrix/1
  Gain/1 -> Product/1
  Constant4/1 -> Sum/2
  Constant3/1 -> Sum1/2
  angle/1 -> Trigonometric Function4/1, Trigonometric Function1/1, Sum1/1, Sum/1
  Trigonometric Function3/1 -> Mux1/2
  Trigonometric Function2/1 -> Mux1/1
  Constant2/1 -> Mux1/3
  Sum/1 -> Trigonometric Function3/1, Trigonometric Function2/1
  Trigonometric Function4/1 -> Mux2/2
  Trigonometric Function1/1 -> Mux2/1
  Constant1/1 -> Mux2/3
  Trigonometric Function6/1 -> Mux3/2
  Trigonometric Function5/1 -> Mux3/1
  Constant5/1 -> Mux3/3
  Sum1/1 -> Trigonometric Function6/1, Trigonometric Function5/1
  Mux1/1 -> Matrix Concatenate/2
  Mux2/1 -> Matrix Concatenate/1
  Mux3/1 -> Matrix Concatenate/3

== system SG_GFOL_2020a/Subsystem1/PQ control/PI_P ==
  er_isat : Inport
  er_P : Inport  Port=2
  Vq : Inport  Port=3
  Divide9 : Product  Inputs=**
  Gain10 : Gain  Gain=-3/2
  Gain11 : Gain  Gain=kp_p_n2
  Gain12 : Gain  Gain=ki_p_n2
  Gain13 : Gain  Gain=ki_p_n2/kp_p_n2
  Integrator3 : Integrator  InitialCondition=Pvsc0
  Sum7 : Sum  Inputs=|++
  Sum8 : Sum  Inputs=|++
  u : Outport  VectorParamsAs1DForOutWhenUnconnected=off
  wires:
  Sum8/1 -> u/1
  Sum7/1 -> Integrator3/1
  Gain12/1 -> Sum7/1
  Gain13/1 -> Sum7/2
  Gain11/1 -> Sum8/1
  er_P/1 -> Gain11/1, Gain12/1
  Integrator3/1 -> Sum8/2
  Vq/1 -> Divide9/2
  Divide9/1 -> Gain10/1
  er_isat/1 -> Divide9/1
  Gain10/1 -> Gain13/1

== system SG_GFOL_2020a/Subsystem1/PQ control/PI_Q ==
  er_isat : Inport
  er_Q : Inport  Port=2
  Vq : Inport  Port=3
  Divide9 : Product  Inputs=**
  Gain10 : Gain  Gain=-3/2
  Gain11 : Gain  Gain=kp_q_n2
  Gain12 : Gain  Gain=ki_q_n2
  Gain13 : Gain  Gain=ki_q_n2/kp_q_n2
  Integrator3 : Integrator
  Sum7 : Sum  Inputs=|++
  Sum8 : Sum  Inputs=|++
  Sum9 : Sum  Inputs=-+|
  u : Outport  VectorParamsAs1DForOutWhenUnconnected=off
  wires:
  Gain10/1 -> Gain13/1
  er_isat/1 -> Divide9/1
  Divide9/1 -> Gain10/1
  Vq/1 -> Divide9/2
  [icd_ref] -> Sum9/2
  [icd_ref_unsat] -> Sum9/1
  Integrator3/1 -> Sum8/2
  er_Q/1 -> Gain12/1, Gain11/1
  Gain11/1 -> Sum8/1
  Gain13/1 -> Sum7/2
  Gain12/1 -> Sum7/1
  Sum7/1 -> Integrator3/1
  Sum8/1 -> u/1

== system SG_GFOL_2020a/Subsystem1/PQ control/Saturation1 ==
  iq_ref : Inport
  id_ref : Inport  Port=2
  Constant8 : Constant  Value=Inom_n2^2
  Gain11 : Gain  Gain=-1
  Math Function : Math  Operator=magnitude^2  SignedPower=on
  Saturation Dynamic : simulink/Discontinuities/Saturation Dynamic  OutMin=[]  OutMax=[]  OutDataTypeStr=Inherit: Same as second input  OutDataType=fixdt(1, 16)  OutScaling=2^-10  DoSatur=off
  Signed Sqrt : Sqrt
  Sum14 : Sum  Inputs=|+-
  Iq_ref_sat : Outport  VectorParamsAs1DForOutWhenUnconnected=off
  wires:
  iq_ref/1 -> Saturation Dynamic/2
  Constant8/1 -> Sum14/1
  Signed Sqrt/1 -> Gain11/1, Saturation Dynamic/1
  Gain11/1 -> Saturation Dynamic/3
  id_ref/1 -> Math Function/1
  Math Function/1 -> Sum14/2
  Saturation Dynamic/1 -> Iq_ref_sat/1
  Sum14/1 -> Signed Sqrt/1

== system SG_GFOL_2020a/G1/Exciter System/SEXS/1st ord transfer fcn windup limiter ==
  note: First order transfer function with windup limiter (non-saturated output)
  In1 : Inport
  Compare To Constant : simulink/Logic and Bit Operations/Compare To Constant  relop=<=  const=Vmax  OutDataTypeStr=boolean
  Compare To Constant1 : simulink/Logic and Bit Operations/Compare To Constant  relop=>=  const=Vmin  OutDataTypeStr=boolean
  OR : Logic  Operator=OR  IconShape=distinctive  AllPortsSameDT=off  OutDataTypeStr=boolean
  Sample and Hold1 : spsSampleandHoldLib/Sample and Hold  ic=0  Ts=0
      settings: LibrarySourceBlock=|
      | sps_lib/Control/Sample and
      | Hold
  Saturation1 : Saturate  UpperLimit=Vmax  LowerLimit=Vmin
  Transfer Fcn (with initial outputs)2 : simulink_extras/Additional Linear/Transfer Fcn (with initial outputs)  N=[Gain]  D=[tau 1]  Y0=y0  U0=y0/Gain
  Out1 : Outport
  wires:
  Sample and Hold1/1 -> Transfer Fcn (with initial outputs)2/1
  Transfer Fcn (with initial outputs)2/1 -> Saturation1/1, Compare To Constant1/1, Compare To Constant/1
  In1/1 -> Sample and Hold1/1
  Compare To Constant/1 -> OR/1
  Compare To Constant1/1 -> OR/2
  OR/1 -> Sample and Hold1/2
  Saturation1/1 -> Out1/1

== system SG_GFOL_2020a/Other blocks (do not use)/PQ/PLL/ParkTransform7 ==
  ABC vector : Inport
  angle : Inport  Port=2
  Constant1 : Constant  Value=1/2
  Constant2 : Constant  Value=1/2
  Constant3 : Constant  Value=2*pi/3
  Constant4 : Constant  Value=2*pi/3
  Constant5 : Constant  Value=1/2
  Gain : Gain  Gain=2/3
  Matrix Concatenate : Concatenate  NumInputs=3  Mode=Multidimensional array  ConcatenateDimension=2
  Mux1 : Mux  Inputs=3
  Mux2 : Mux  Inputs=3
  Mux3 : Mux  Inputs=3
  Product : Product  Multiplication=Matrix(*)  RndMeth=Zero
  Sum : Sum  Inputs=|+-
  Sum1 : Sum  Inputs=|++
  Trigonometric Function1 : Trigonometry  Operator=cos
  Trigonometric Function2 : Trigonometry  Operator=cos
  Trigonometric Function3 : Trigonometry
  Trigonometric Function4 : Trigonometry
  Trigonometric Function5 : Trigonometry  Operator=cos
  Trigonometric Function6 : Trigonometry
  Matrix : Outport
  wires:
  Mux3/1 -> Matrix Concatenate/3
  Mux2/1 -> Matrix Concatenate/1
  Mux1/1 -> Matrix Concatenate/2
  Sum1/1 -> Trigonometric Function5/1, Trigonometric Function6/1
  Constant5/1 -> Mux3/3
  Trigonometric Function5/1 -> Mux3/1
  Trigonometric Function6/1 -> Mux3/2
  Constant1/1 -> Mux2/3
  Trigonometric Function1/1 -> Mux2/1
  Trigonometric Function4/1 -> Mux2/2
  Sum/1 -> Trigonometric Function2/1, Trigonometric Function3/1
  Constant2/1 -> Mux1/3
  Trigonometric Function2/1 -> Mux1/1
  Trigonometric Function3/1 -> Mux1/2
  angle/1 -> Sum/1, Sum1/1, Trigonometric Function1/1, Trigonometric Function4/1
  Constant3/1 -> Sum1/2
  Constant4/1 -> Sum/2
  Gain/1 -> Product/1
  Product/1 -> Matrix/1
  ABC vector/1 -> Product/2
  Matrix Concatenate/1 -> Gain/1
